simulink model "wpt"  (R2022b)
settings: Solver=VariableStepAuto  StartTime=0.0  StopTime=0.1  RelTol=1e-3
undefined symbols (not defined in the file): Ion, Lithium
libraries: spsDiodeLib x8, spsSeriesRLCBranchLib x6, spsVoltageMeasurementLib x6, spsCurrentMeasurementLib x5, spsPowerPhasorLib x5, spsIGBTDiodeLib x4, spsACVoltageSourceLib x1, spsBatteryLib x1, spsPWMGeneratorDCDCLib x1, spsMutualInductanceLib x1, spspowerguiLib x1
settings Model: Creator=ahmed  LastModifiedBy=ahmed

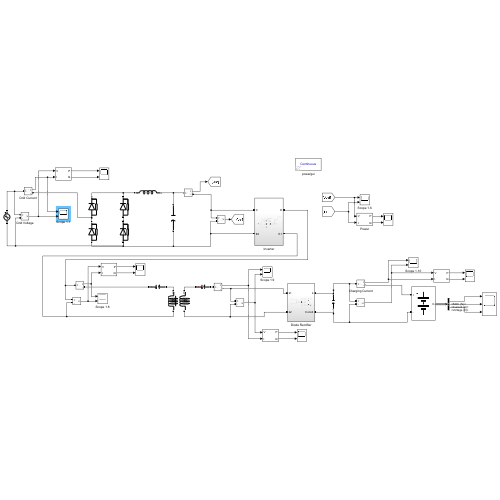
[thumbnail: Simulink's stored preview of the top-level diagram]
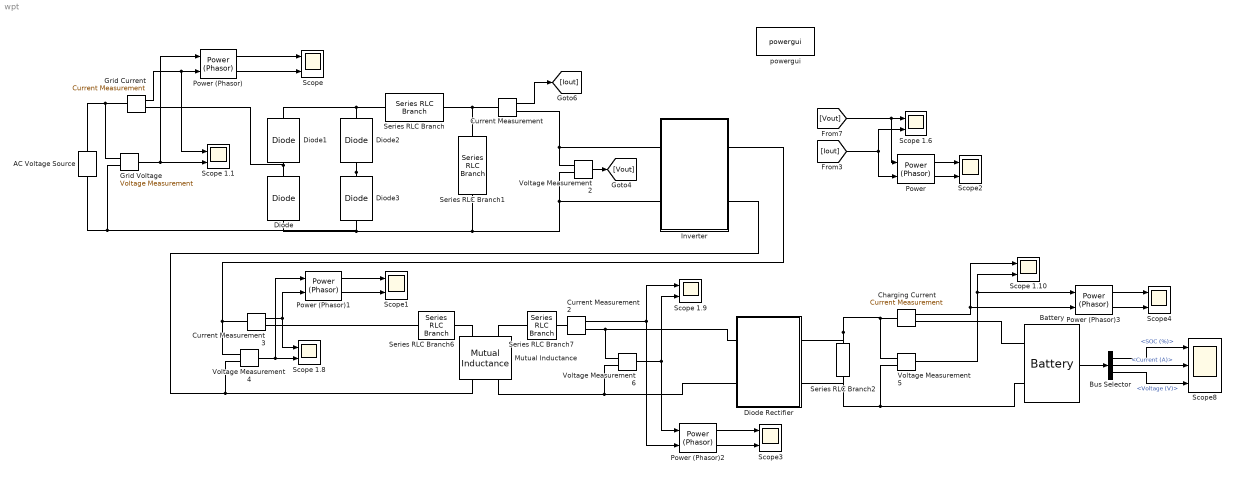
== system wpt ==
  AC Voltage Source : spsACVoltageSourceLib/AC Voltage Source  Amplitude=325  Phase=0  Frequency=50  SampleTime=0  Measurements=None  BusType=swing  Pref=10e3  Qref=0  Qmin=-inf  Qmax=+inf
  Battery : spsBatteryLib/Battery  BatType=Lithium-Ion  ShowTempParam=off  ThermalPreset=no  ShowAgeParam=off  NomV=48  NomQ=150  SOC=90  Batt_Tr=0.1  PresetModel=on  MaxQ=150  MinV=36  FullV=55.8714  Dis_rate=65.2174  R=0.0032  Normal_OP=135.6522  expZone="[51.8585      7.36957]"  current=[6.5 13 32.5]  Units=Time  Tci=20  NomT=20  T2=-30  MaxQ2=4.8  FullV2=7.1  Normal_OP2=5.655  expZone2="[6.58           1]"  Rca=0.6  ti=2000  Dp=0  Neq0=0  Tsim=1e6  Ta1=25  Qeol=5.4*0.9  Reol=0.013333*1.2  Char_age=[2.3478, 3]  Dis_age=[2.3478, 10]  N1=1500  N2=10500  N3=1000  N4=1400  Ta2=45  N5=950
  Bus Selector : BusSelector  OutputSignals=SOC (%),Current (A),Voltage (V)
  Charging Current : spsCurrentMeasurementLib/Current Measurement  PhasorSimulation=off  OutputType=Complex  PSBequivalent=0
  Current Measurement : spsCurrentMeasurementLib/Current Measurement  PhasorSimulation=off  OutputType=Complex  PSBequivalent=0
  Current Measurement2 : spsCurrentMeasurementLib/Current Measurement  PhasorSimulation=off  OutputType=Complex  PSBequivalent=0
  Current Measurement3 : spsCurrentMeasurementLib/Current Measurement  PhasorSimulation=off  OutputType=Complex  PSBequivalent=0
  Diode{,1..3} (4 alike) : spsDiodeLib/Diode  Ron=0.001  Lon=0  Vf=0.8  IC=0  UseSnubber=0  Rs=500  Cs=250e-9  Measurements=off
  Diode Rectifier : Subsystem
  Grid Current : spsCurrentMeasurementLib/Current Measurement  PhasorSimulation=off  OutputType=Complex  PSBequivalent=0
  Grid Voltage : spsVoltageMeasurementLib/Voltage Measurement  PhasorSimulation=off  OutputType=Complex  PSBequivalent=0
  Inverter : Subsystem
  Mutual Inductance : spsMutualInductanceLib/Mutual Inductance  LConnTagsString=a|b  RConnTagsString=A|B  TypeOfMutual=Two or three windings with equal mutual terms  NumberOfWindings=3  SelfImpedance1=[1e-3 137.804e-6]  SelfImpedance2=[ 1e-3 137.804e-6 ]  ThreeWindings=off  SelfImpedance3=[ 1.1 1.1e-03]  MutualImpedance=[0 36.236e-6 ]  InductanceMatrix="[1.0 0.9  0.9 ;  0.9 1.0  0.9;  0.9 0.9 1.0 ] * 1e-3"  ResistanceMatrix="[1.0 0.9  0.9 ;  0.9 1.0  0.9;  0.9 0.9 1.0 ]"  Measurements=None
  Power : spsPowerPhasorLib/Power (Phasor)
  Power (Phasor){,1..3} (4 alike) : spsPowerPhasorLib/Power (Phasor)
  Scope{,1..4} (5 alike) : Scope  NumInputPorts=2
  Scope 1.{1,6,8..10} (5 alike) : Scope  NumInputPorts=2
  Scope8 : Scope  NumInputPorts=3
  Series RLC Branch : spsSeriesRLCBranchLib/Series RLC Branch  LConnTagsString=__new0  RConnTagsString=__new0  BranchType=L  Resistance=1  Inductance=0.3e-3  SetiL0=off  InitialCurrent=0  Capacitance=1e-6  Setx0=off  InitialVoltage=0  Measurements=None
  Series RLC Branch1 : spsSeriesRLCBranchLib/Series RLC Branch  LConnTagsString=__new0  RConnTagsString=__new0  BranchType=C  Resistance=1  Inductance=1e-3  SetiL0=off  InitialCurrent=0  Capacitance=2000e-6  Setx0=off  InitialVoltage=0  Measurements=None
  Series RLC Branch2 : spsSeriesRLCBranchLib/Series RLC Branch  LConnTagsString=__new0  RConnTagsString=__new0  BranchType=C  Resistance=1  Inductance=1e-3  SetiL0=off  InitialCurrent=0  Capacitance=300e-6  Setx0=off  InitialVoltage=0  Measurements=None
  Series RLC Branch6 : spsSeriesRLCBranchLib/Series RLC Branch  LConnTagsString=__new0  RConnTagsString=__new0  BranchType=C  Resistance=1  Inductance=1e-3  SetiL0=off  InitialCurrent=0  Capacitance=39.093e-9  Setx0=off  InitialVoltage=0  Measurements=None
  Series RLC Branch7 : spsSeriesRLCBranchLib/Series RLC Branch  LConnTagsString=__new0  RConnTagsString=__new0  BranchType=C  Resistance=1  Inductance=1e-3  SetiL0=off  InitialCurrent=0  Capacitance=25.43e-9  Setx0=off  InitialVoltage=0  Measurements=None
  Voltage Measurement{2,4..6} (4 alike) : spsVoltageMeasurementLib/Voltage Measurement  PhasorSimulation=off  OutputType=Complex  PSBequivalent=0
  powergui : spspowerguiLib/powergui  Priority=1  SimulationMode=Continuous  SampleTime=1e-6  frequency=60  Iterations=50  frequencyindice=0  Pbase=100e6  ErrMax=1e-4  UnitsV=kV  UnitsW=MW  buscounter=0  FunctionMessages=off  echomessages=off  EnableUseOfTLC=off  CurrentSourceSwitches=off  DisableSnubberDevices=off  DisableRonSwitches=off  DisableVfSwitches=off  DisplayEquations=off  AutomaticDiscreteSolvers=off  SolverType=Tustin/Backward Euler (TBE)  Interpol=off  ExternalGateDelay=off  methode=off  Ts=100  x0status=blocks  SPID=on  SwTol=0  HookPort=off  NonlinearTolerance=1e-4  nMaxIteration=100  ContinueOnMaxIteration=off  RestoreLinks=warning  ResistiveCurrentMeasurement=off  Frange=[0:2:500]  Ylog=off  Xlog=on  ShowGrid=off  save=off  variable=ZData  structure=0  ZoomFFT=off  StartTime=0.0  cycles=1  DisplayStyle=1  fundamental=60  FreqAxis=off  MaxFrequency=1000  frequencyindicesteady=1  RmsSteady=1  display=off
  wires:
  Power (Phasor)/2 -> Scope/2
  Power (Phasor)/1 -> Scope/1
  Grid Voltage/1 -> Scope 1.1/2, Power (Phasor)/1
  Current Measurement/1 -> [Iout]
  Voltage Measurement2/1 -> [Vout]
  Power/1 -> Scope2/1
  [Vout] -> Scope 1.6/1, Power/1
  Power/2 -> Scope2/2
  [Iout] -> Scope 1.6/2, Power/2
  Power (Phasor)2/1 -> Scope3/1
  Bus Selector/3 -> Scope8/3  "<Voltage (V)>"
  Battery/1 -> Bus Selector/1
  Bus Selector/2 -> Scope8/2  "<Current (A)>"
  Charging Current/1 -> Scope 1.10/1, Power (Phasor)3/2
  Power (Phasor)3/2 -> Scope4/2
  Voltage Measurement5/1 -> Scope 1.10/2, Power (Phasor)3/1
  Power (Phasor)2/2 -> Scope3/2
  Power (Phasor)1/2 -> Scope1/2
  Current Measurement2/1 -> Scope 1.9/1, Power (Phasor)2/2
  Voltage Measurement6/1 -> Scope 1.9/2, Power (Phasor)2/1
  Power (Phasor)1/1 -> Scope1/1
  Voltage Measurement4/1 -> Scope 1.8/2, Power (Phasor)1/1
  Bus Selector/1 -> Scope8/1  "<SOC (%)>"
  Power (Phasor)3/1 -> Scope4/1
  Current Measurement3/1 -> Scope 1.8/1, Power (Phasor)1/2
  Grid Current/1 -> Scope 1.1/1, Power (Phasor)/2
  connections:
  AC Voltage Source/RConn1 -- Grid Voltage/LConn1 -- Grid Current/LConn1
  Diode1/LConn1 -- Grid Current/RConn1 -- Diode/RConn1
  Diode3/RConn1 -- Grid Voltage/LConn2 -- AC Voltage Source/LConn1 -- Diode2/LConn1
  Diode2/RConn1 -- Series RLC Branch/LConn1 -- Diode1/RConn1
  Diode/LConn1 -- Voltage Measurement2/LConn2 -- Inverter/LConn2 -- Series RLC Branch1/RConn1 -- Diode3/LConn1
  Series RLC Branch1/LConn1 -- Current Measurement/LConn1 -- Series RLC Branch/RConn1
  Current Measurement/RConn1 -- Voltage Measurement2/LConn1 -- Inverter/LConn1
  Mutual Inductance/RConn1 -- Voltage Measurement4/LConn2 -- Inverter/RConn2
  Mutual Inductance/RConn2 -- Diode Rectifier/LConn2 -- Voltage Measurement6/LConn2
  Series RLC Branch2/RConn1 -- Voltage Measurement5/LConn2 -- Battery/LConn2 -- Diode Rectifier/RConn2
  Voltage Measurement6/LConn1 -- Diode Rectifier/LConn1 -- Current Measurement2/RConn1
  Charging Current/LConn1 -- Diode Rectifier/RConn1 -- Series RLC Branch2/LConn1 -- Voltage Measurement5/LConn1
  Current Measurement2/LConn1 -- Series RLC Branch7/RConn1
  Mutual Inductance/LConn2 -- Series RLC Branch7/LConn1
  Mutual Inductance/LConn1 -- Series RLC Branch6/RConn1
  Battery/LConn1 -- Charging Current/RConn1
  Current Measurement3/LConn1 -- Voltage Measurement4/LConn1 -- Inverter/RConn1
  Series RLC Branch6/LConn1 -- Current Measurement3/RConn1

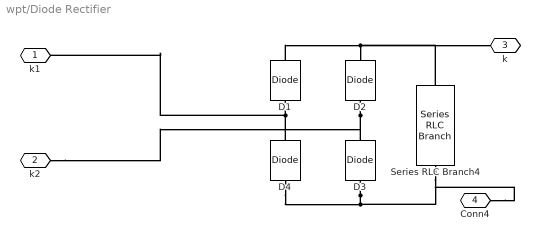
== system wpt/Diode Rectifier ==
  D{1..4} (4 alike) : spsDiodeLib/Diode  Ron=0.001  Lon=0  Vf=0.8  IC=0  UseSnubber=0  Rs=500  Cs=250e-9  Measurements=off
  Series RLC Branch4 : spsSeriesRLCBranchLib/Series RLC Branch  LConnTagsString=__new0  RConnTagsString=__new0  BranchType=C  Resistance=1  Inductance=1e-3  SetiL0=off  InitialCurrent=0  Capacitance=100e-6  Setx0=off  InitialVoltage=0  Measurements=None
  k1 : PMIOPort  Side=Left
  k2 : PMIOPort  Port=2  Side=Left
  k : PMIOPort  Port=3  Side=Right
  Conn4 : PMIOPort  Port=4  Side=Right
  connections:
  D3/LConn1 -- D4/LConn1 -- Conn4/RConn1 -- Series RLC Branch4/RConn1
  D2/LConn1 -- D3/RConn1 -- k2/RConn1
  D2/RConn1 -- D1/RConn1 -- Series RLC Branch4/LConn1 -- k/RConn1
  D1/LConn1 -- D4/RConn1 -- k1/RConn1

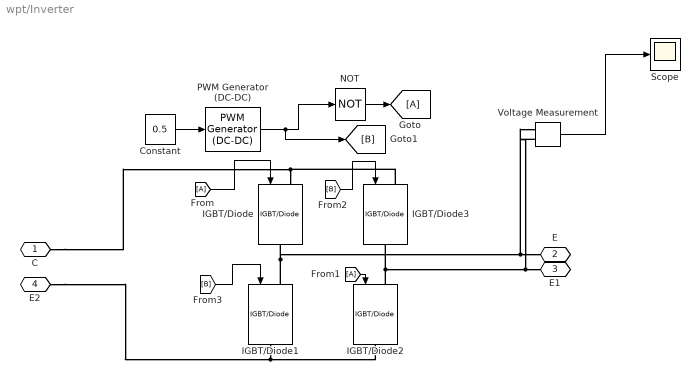
== system wpt/Inverter ==
  Constant : Constant  Value=0.5
  From : From
  From1 : From
  Goto : Goto
  IGBT/Diode{,1..3} (4 alike) : spsIGBTDiodeLib/IGBT//Diode  Ron=1e-3  Rs=1e5  Cs=inf  Measurements=off
  NOT : Logic  Operator=NOT  IconShape=distinctive  AllPortsSameDT=off  OutDataTypeStr=boolean
  PWM Generator (DC-DC) : spsPWMGeneratorDCDCLib/PWM Generator (DC-DC)  Fsw=85000  Ts=0
  Scope : Scope
  Voltage Measurement : spsVoltageMeasurementLib/Voltage Measurement  PhasorSimulation=off  OutputType=Complex  PSBequivalent=0
  C : PMIOPort  Side=Left
  E : PMIOPort  Port=2  Side=Right
  E1 : PMIOPort  Port=3  Side=Right
  E2 : PMIOPort  Port=4  Side=Left
  wires:
  NOT/1 -> Goto/1
  From1/1 -> IGBT/Diode2/1
  Constant/1 -> PWM Generator (DC-DC)/1
  [B] -> IGBT/Diode1/1
  From/1 -> IGBT/Diode/1
  PWM Generator (DC-DC)/1 -> [B], NOT/1
  [B] -> IGBT/Diode3/1
  Voltage Measurement/1 -> Scope/1
  connections:
  IGBT/Diode2/LConn1 -- Voltage Measurement/LConn2 -- E1/RConn1 -- IGBT/Diode3/RConn1
  IGBT/Diode1/RConn1 -- E2/RConn1 -- IGBT/Diode2/RConn1
  IGBT/Diode3/LConn1 -- C/RConn1 -- IGBT/Diode/LConn1
  IGBT/Diode1/LConn1 -- Voltage Measurement/LConn1 -- E/RConn1 -- IGBT/Diode/RConn1
